simulink model "gm_minutiaeextraction_21821"  (R2018b)
settings: Solver=FixedStepDiscrete  StartTime=0.0  StopTime=10  RelTol=1e-3
undefined symbols (not defined in the file or in its folder): gray
libraries: hdlsllib x4, visionsources x1, dspmtrx3 x1
(part 7 of 7)

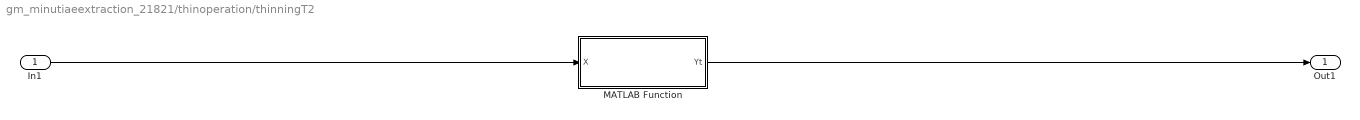
== system gm_minutiaeextraction_21821/thinoperation/thinningT2 ==
  In1 : Inport
  MATLAB Function : MATLAB Function  TreatAsAtomicUnit=on
  Out1 : Outport
  wires:
  MATLAB Function/1(Yt) -> Out1/1
  In1/1 -> MATLAB Function/1(X)

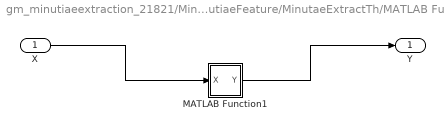
== system gm_minutiaeextraction_21821/MinutiaeFeature/MinutaeExtractTh/MATLAB Function1 ==
  X : Inport  OutDataTypeStr=boolean  PortDimensions=[128,64]  SampleTime=0.1
  MATLAB Function1 : MATLAB Function  TreatAsAtomicUnit=on
  Y : Outport
  wires:
  X/1 -> MATLAB Function1/1(X)
  MATLAB Function1/1(Y) -> Y/1

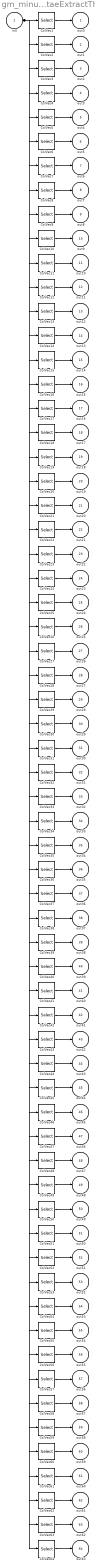
== system gm_minutiaeextraction_21821/MinutiaeFeature/MinutaeExtractTh/t ==
  in0 : Inport
  ColVec1 : Selector  NumberOfDimensions=2  IndexOptions=Select all,Index vector (dialog)  Indices=1,1  OutputSizes=1,1
  ColVec10 : Selector  NumberOfDimensions=2  IndexOptions=Select all,Index vector (dialog)  Indices=1,10  OutputSizes=1,1
  ColVec11 : Selector  NumberOfDimensions=2  IndexOptions=Select all,Index vector (dialog)  Indices=1,11  OutputSizes=1,1
  ColVec12 : Selector  NumberOfDimensions=2  IndexOptions=Select all,Index vector (dialog)  Indices=1,12  OutputSizes=1,1
  ColVec13 : Selector  NumberOfDimensions=2  IndexOptions=Select all,Index vector (dialog)  Indices=1,13  OutputSizes=1,1
  ColVec14 : Selector  NumberOfDimensions=2  IndexOptions=Select all,Index vector (dialog)  Indices=1,14  OutputSizes=1,1
  ColVec15 : Selector  NumberOfDimensions=2  IndexOptions=Select all,Index vector (dialog)  Indices=1,15  OutputSizes=1,1
  ColVec16 : Selector  NumberOfDimensions=2  IndexOptions=Select all,Index vector (dialog)  Indices=1,16  OutputSizes=1,1
  ColVec17 : Selector  NumberOfDimensions=2  IndexOptions=Select all,Index vector (dialog)  Indices=1,17  OutputSizes=1,1
  ColVec18 : Selector  NumberOfDimensions=2  IndexOptions=Select all,Index vector (dialog)  Indices=1,18  OutputSizes=1,1
  ColVec19 : Selector  NumberOfDimensions=2  IndexOptions=Select all,Index vector (dialog)  Indices=1,19  OutputSizes=1,1
  ColVec2 : Selector  NumberOfDimensions=2  IndexOptions=Select all,Index vector (dialog)  Indices=1,2  OutputSizes=1,1
  ColVec20 : Selector  NumberOfDimensions=2  IndexOptions=Select all,Index vector (dialog)  Indices=1,20  OutputSizes=1,1
  ColVec21 : Selector  NumberOfDimensions=2  IndexOptions=Select all,Index vector (dialog)  Indices=1,21  OutputSizes=1,1
  ColVec22 : Selector  NumberOfDimensions=2  IndexOptions=Select all,Index vector (dialog)  Indices=1,22  OutputSizes=1,1
  ColVec23 : Selector  NumberOfDimensions=2  IndexOptions=Select all,Index vector (dialog)  Indices=1,23  OutputSizes=1,1
  ColVec24 : Selector  NumberOfDimensions=2  IndexOptions=Select all,Index vector (dialog)  Indices=1,24  OutputSizes=1,1
  ColVec25 : Selector  NumberOfDimensions=2  IndexOptions=Select all,Index vector (dialog)  Indices=1,25  OutputSizes=1,1
  ColVec26 : Selector  NumberOfDimensions=2  IndexOptions=Select all,Index vector (dialog)  Indices=1,26  OutputSizes=1,1
  ColVec27 : Selector  NumberOfDimensions=2  IndexOptions=Select all,Index vector (dialog)  Indices=1,27  OutputSizes=1,1
  ColVec28 : Selector  NumberOfDimensions=2  IndexOptions=Select all,Index vector (dialog)  Indices=1,28  OutputSizes=1,1
  ColVec29 : Selector  NumberOfDimensions=2  IndexOptions=Select all,Index vector (dialog)  Indices=1,29  OutputSizes=1,1
  ColVec3 : Selector  NumberOfDimensions=2  IndexOptions=Select all,Index vector (dialog)  Indices=1,3  OutputSizes=1,1
  ColVec30 : Selector  NumberOfDimensions=2  IndexOptions=Select all,Index vector (dialog)  Indices=1,30  OutputSizes=1,1
  ColVec31 : Selector  NumberOfDimensions=2  IndexOptions=Select all,Index vector (dialog)  Indices=1,31  OutputSizes=1,1
  ColVec32 : Selector  NumberOfDimensions=2  IndexOptions=Select all,Index vector (dialog)  Indices=1,32  OutputSizes=1,1
  ColVec33 : Selector  NumberOfDimensions=2  IndexOptions=Select all,Index vector (dialog)  Indices=1,33  OutputSizes=1,1
  ColVec34 : Selector  NumberOfDimensions=2  IndexOptions=Select all,Index vector (dialog)  Indices=1,34  OutputSizes=1,1
  ColVec35 : Selector  NumberOfDimensions=2  IndexOptions=Select all,Index vector (dialog)  Indices=1,35  OutputSizes=1,1
  ColVec36 : Selector  NumberOfDimensions=2  IndexOptions=Select all,Index vector (dialog)  Indices=1,36  OutputSizes=1,1
  ColVec37 : Selector  NumberOfDimensions=2  IndexOptions=Select all,Index vector (dialog)  Indices=1,37  OutputSizes=1,1
  ColVec38 : Selector  NumberOfDimensions=2  IndexOptions=Select all,Index vector (dialog)  Indices=1,38  OutputSizes=1,1
  ColVec39 : Selector  NumberOfDimensions=2  IndexOptions=Select all,Index vector (dialog)  Indices=1,39  OutputSizes=1,1
  ColVec4 : Selector  NumberOfDimensions=2  IndexOptions=Select all,Index vector (dialog)  Indices=1,4  OutputSizes=1,1
  ColVec40 : Selector  NumberOfDimensions=2  IndexOptions=Select all,Index vector (dialog)  Indices=1,40  OutputSizes=1,1
  ColVec41 : Selector  NumberOfDimensions=2  IndexOptions=Select all,Index vector (dialog)  Indices=1,41  OutputSizes=1,1
  ColVec42 : Selector  NumberOfDimensions=2  IndexOptions=Select all,Index vector (dialog)  Indices=1,42  OutputSizes=1,1
  ColVec43 : Selector  NumberOfDimensions=2  IndexOptions=Select all,Index vector (dialog)  Indices=1,43  OutputSizes=1,1
  ColVec44 : Selector  NumberOfDimensions=2  IndexOptions=Select all,Index vector (dialog)  Indices=1,44  OutputSizes=1,1
  ColVec45 : Selector  NumberOfDimensions=2  IndexOptions=Select all,Index vector (dialog)  Indices=1,45  OutputSizes=1,1
  ColVec46 : Selector  NumberOfDimensions=2  IndexOptions=Select all,Index vector (dialog)  Indices=1,46  OutputSizes=1,1
  ColVec47 : Selector  NumberOfDimensions=2  IndexOptions=Select all,Index vector (dialog)  Indices=1,47  OutputSizes=1,1
  ColVec48 : Selector  NumberOfDimensions=2  IndexOptions=Select all,Index vector (dialog)  Indices=1,48  OutputSizes=1,1
  ColVec49 : Selector  NumberOfDimensions=2  IndexOptions=Select all,Index vector (dialog)  Indices=1,49  OutputSizes=1,1
  ColVec5 : Selector  NumberOfDimensions=2  IndexOptions=Select all,Index vector (dialog)  Indices=1,5  OutputSizes=1,1
  ColVec50 : Selector  NumberOfDimensions=2  IndexOptions=Select all,Index vector (dialog)  Indices=1,50  OutputSizes=1,1
  ColVec51 : Selector  NumberOfDimensions=2  IndexOptions=Select all,Index vector (dialog)  Indices=1,51  OutputSizes=1,1
  ColVec52 : Selector  NumberOfDimensions=2  IndexOptions=Select all,Index vector (dialog)  Indices=1,52  OutputSizes=1,1
  ColVec53 : Selector  NumberOfDimensions=2  IndexOptions=Select all,Index vector (dialog)  Indices=1,53  OutputSizes=1,1
  ColVec54 : Selector  NumberOfDimensions=2  IndexOptions=Select all,Index vector (dialog)  Indices=1,54  OutputSizes=1,1
  ColVec55 : Selector  NumberOfDimensions=2  IndexOptions=Select all,Index vector (dialog)  Indices=1,55  OutputSizes=1,1
  ColVec56 : Selector  NumberOfDimensions=2  IndexOptions=Select all,Index vector (dialog)  Indices=1,56  OutputSizes=1,1
  ColVec57 : Selector  NumberOfDimensions=2  IndexOptions=Select all,Index vector (dialog)  Indices=1,57  OutputSizes=1,1
  ColVec58 : Selector  NumberOfDimensions=2  IndexOptions=Select all,Index vector (dialog)  Indices=1,58  OutputSizes=1,1
  ColVec59 : Selector  NumberOfDimensions=2  IndexOptions=Select all,Index vector (dialog)  Indices=1,59  OutputSizes=1,1
  ColVec6 : Selector  NumberOfDimensions=2  IndexOptions=Select all,Index vector (dialog)  Indices=1,6  OutputSizes=1,1
  ColVec60 : Selector  NumberOfDimensions=2  IndexOptions=Select all,Index vector (dialog)  Indices=1,60  OutputSizes=1,1
  ColVec61 : Selector  NumberOfDimensions=2  IndexOptions=Select all,Index vector (dialog)  Indices=1,61  OutputSizes=1,1
  ColVec62 : Selector  NumberOfDimensions=2  IndexOptions=Select all,Index vector (dialog)  Indices=1,62  OutputSizes=1,1
  ColVec63 : Selector  NumberOfDimensions=2  IndexOptions=Select all,Index vector (dialog)  Indices=1,63  OutputSizes=1,1
  ColVec64 : Selector  NumberOfDimensions=2  IndexOptions=Select all,Index vector (dialog)  Indices=1,64  OutputSizes=1,1
  ColVec7 : Selector  NumberOfDimensions=2  IndexOptions=Select all,Index vector (dialog)  Indices=1,7  OutputSizes=1,1
  ColVec8 : Selector  NumberOfDimensions=2  IndexOptions=Select all,Index vector (dialog)  Indices=1,8  OutputSizes=1,1
  ColVec9 : Selector  NumberOfDimensions=2  IndexOptions=Select all,Index vector (dialog)  Indices=1,9  OutputSizes=1,1
  out0 : Outport
  out1 : Outport  Port=2
  out2 : Outport  Port=3
  out3 : Outport  Port=4
  out4 : Outport  Port=5
  out5 : Outport  Port=6
  out6 : Outport  Port=7
  out7 : Outport  Port=8
  out8 : Outport  Port=9
  out9 : Outport  Port=10
  out10 : Outport  Port=11
  out11 : Outport  Port=12
  out12 : Outport  Port=13
  out13 : Outport  Port=14
  out14 : Outport  Port=15
  out15 : Outport  Port=16
  out16 : Outport  Port=17
  out17 : Outport  Port=18
  out18 : Outport  Port=19
  out19 : Outport  Port=20
  out20 : Outport  Port=21
  out21 : Outport  Port=22
  out22 : Outport  Port=23
  out23 : Outport  Port=24
  out24 : Outport  Port=25
  out25 : Outport  Port=26
  out26 : Outport  Port=27
  out27 : Outport  Port=28
  out28 : Outport  Port=29
  out29 : Outport  Port=30
  out30 : Outport  Port=31
  out31 : Outport  Port=32
  out32 : Outport  Port=33
  out33 : Outport  Port=34
  out34 : Outport  Port=35
  out35 : Outport  Port=36
  out36 : Outport  Port=37
  out37 : Outport  Port=38
  out38 : Outport  Port=39
  out39 : Outport  Port=40
  out40 : Outport  Port=41
  out41 : Outport  Port=42
  out42 : Outport  Port=43
  out43 : Outport  Port=44
  out44 : Outport  Port=45
  out45 : Outport  Port=46
  out46 : Outport  Port=47
  out47 : Outport  Port=48
  out48 : Outport  Port=49
  out49 : Outport  Port=50
  out50 : Outport  Port=51
  out51 : Outport  Port=52
  out52 : Outport  Port=53
  out53 : Outport  Port=54
  out54 : Outport  Port=55
  out55 : Outport  Port=56
  out56 : Outport  Port=57
  out57 : Outport  Port=58
  out58 : Outport  Port=59
  out59 : Outport  Port=60
  out60 : Outport  Port=61
  out61 : Outport  Port=62
  out62 : Outport  Port=63
  out63 : Outport  Port=64
  wires:
  in0/1 -> ColVec1/1, ColVec2/1, ColVec3/1, ColVec4/1, ColVec5/1, ColVec6/1, ColVec7/1, ColVec8/1, ColVec9/1, ColVec10/1, ColVec11/1, ColVec12/1, ColVec13/1, ColVec14/1, ColVec15/1, ColVec16/1, ColVec17/1, ColVec18/1, ColVec19/1, ColVec20/1, ColVec21/1, ColVec22/1, ColVec23/1, ColVec24/1, ColVec25/1, ColVec26/1, ColVec27/1, ColVec28/1, ColVec29/1, ColVec30/1, ColVec31/1, ColVec32/1, ColVec33/1, ColVec34/1, ColVec35/1, ColVec36/1, ColVec37/1, ColVec38/1, ColVec39/1, ColVec40/1, ColVec41/1, ColVec42/1, ColVec43/1, ColVec44/1, ColVec45/1, ColVec46/1, ColVec47/1, ColVec48/1, ColVec49/1, ColVec50/1, ColVec51/1, ColVec52/1, ColVec53/1, ColVec54/1, ColVec55/1, ColVec56/1, ColVec57/1, ColVec58/1, ColVec59/1, ColVec60/1, ColVec61/1, ColVec62/1, ColVec63/1, ColVec64/1
  ColVec1/1 -> out0/1
  ColVec2/1 -> out1/1
  ColVec3/1 -> out2/1
  ColVec4/1 -> out3/1
  ColVec5/1 -> out4/1
  ColVec6/1 -> out5/1
  ColVec7/1 -> out6/1
  ColVec8/1 -> out7/1
  ColVec9/1 -> out8/1
  ColVec10/1 -> out9/1
  ColVec11/1 -> out10/1
  ColVec12/1 -> out11/1
  ColVec13/1 -> out12/1
  ColVec14/1 -> out13/1
  ColVec15/1 -> out14/1
  ColVec16/1 -> out15/1
  ColVec17/1 -> out16/1
  ColVec18/1 -> out17/1
  ColVec19/1 -> out18/1
  ColVec20/1 -> out19/1
  ColVec21/1 -> out20/1
  ColVec22/1 -> out21/1
  ColVec23/1 -> out22/1
  ColVec24/1 -> out23/1
  ColVec25/1 -> out24/1
  ColVec26/1 -> out25/1
  ColVec27/1 -> out26/1
  ColVec28/1 -> out27/1
  ColVec29/1 -> out28/1
  ColVec30/1 -> out29/1
  ColVec31/1 -> out30/1
  ColVec32/1 -> out31/1
  ColVec33/1 -> out32/1
  ColVec34/1 -> out33/1
  ColVec35/1 -> out34/1
  ColVec36/1 -> out35/1
  ColVec37/1 -> out36/1
  ColVec38/1 -> out37/1
  ColVec39/1 -> out38/1
  ColVec40/1 -> out39/1
  ColVec41/1 -> out40/1
  ColVec42/1 -> out41/1
  ColVec43/1 -> out42/1
  ColVec44/1 -> out43/1
  ColVec45/1 -> out44/1
  ColVec46/1 -> out45/1
  ColVec47/1 -> out46/1
  ColVec48/1 -> out47/1
  ColVec49/1 -> out48/1
  ColVec50/1 -> out49/1
  ColVec51/1 -> out50/1
  ColVec52/1 -> out51/1
  ColVec53/1 -> out52/1
  ColVec54/1 -> out53/1
  ColVec55/1 -> out54/1
  ColVec56/1 -> out55/1
  ColVec57/1 -> out56/1
  ColVec58/1 -> out57/1
  ColVec59/1 -> out58/1
  ColVec60/1 -> out59/1
  ColVec61/1 -> out60/1
  ColVec62/1 -> out61/1
  ColVec63/1 -> out62/1
  ColVec64/1 -> out63/1

== matlab function gm_minutiaeextraction_21821/MATLAB Function2 ==
  data: u input; y output
function y = fcn(u)
%#codegen
%i = rgb2gray(u);
b = u(100:227,150:213);
y = imbinarize(b);
%y = y(100:227,150:213);
%y = imbinarize(r);

== matlab function gm_minutiaeextraction_21821/thinoperation/thinningT2/MATLAB Function ==
  data: X input; Yt output
function Yt=thinningTh(X)
%img = imread ('2_4.jpg'); 
%Xr = rgb2gray(img);
%%%X = imbinarize(Xr);
%X = X(1:128,1:64);
[M,N]=size(X);
Yt = false(M,N);
Y=false(M,N,20);
Z=false(M,N,20);
Y(:,:,1)=X;
Z(:,:,1)=X;
for k=2:20
    Y(:,:,k)=Y(:,:,k-1);
    for i=2:M-1
        for j=2:N-1
            y11=Y(i-1,j-1,k);
            y12=Y(i-1,j,k);
            y13=Y(i-1,j+1,k);
            y21=Y(i,j-1,k);
            y22=Y(i,j,k);
            y23=Y(i,j+1,k);
            y31=Y(i+1,j-1,k);
            y32=Y(i+1,j,k);
            y33=Y(i+1,j+1,k);
            if y22==0
                if y11==1&&y12==1&&y13==1&&y31==0&&y32==0&&y33==0
                    Y(i,j,k)=1;
                elseif y11==1&&y13==0&&y21==1&&y23==0&&y31==1&&y33==0
                    Y(i,j,k)=1;
                elseif y11==0&&y12==0&&y13==0&&y31==1&&y32==1&&y33==1
                    Y(i,j,k)=1;
                elseif y11==0&&y13==1&&y21==0&&y23==1&&y31==0&&y33==1
                    Y(i,j,k)=1;
                elseif y12==1&&y13==1&&y21==0&&y23==1&&y32==0
                    Y(i,j,k)=1;
                elseif y11==1&&y12==1&&y21==1&&y23==0&&y32==0
                    Y(i,j,k)=1;
                elseif y12==0&&y21==1&&y23==0&&y31==1&&y21==1
                    Y(i,j,k)=1;
                elseif y12==0&&y21==0&&y23==1&&y32==1&&y33==1
                    Y(i,j,k)=1;
                    %extra
                elseif y11==0&&y12==0&&y23==1&&y31==1&&y32==1&&y33==1
                    Y(i,j,k)=1;
                end
            else
            end
        end
    end
%    Y(:,:,k)= Y(:,:,k-1);
     if Y(:,:,k)==Y(:,:,k-1)
%         break;
     end
end
Yt=Y(:,:,k);
%figure;
%imshow(Y);

== matlab function gm_minutiaeextraction_21821/MinutiaeFeature/MinutaeExtractTh/MATLAB Function1/MATLAB Function1 ==
  data: X input; Y output
function Y=minuextractT(X)
%img = imread ('101_7.tif'); 
%Xr = rgb2gray(img);
%Xt = imbinarize(img);
%X=~bwmorph(Xt,'thin',Inf);
[M,N]=size(X);
%mi(:,:)=X;
Y=false(M,N);
Y(:,:)=X;
%[M,N]=size(X);
mi=false(M,N);

for i=2:M-1
    for j=2:N-1
        % * * * y11 y12 y13
        % * @ * y21 y22 y23
        % * * * y31 y32 y33
        y11=Y(i-1,j-1);
        y12=Y(i-1,j);
        y13=Y(i-1,j+1);
        y21=Y(i,j-1);
        y22=Y(i,j);
        y23=Y(i,j+1);
        y31=Y(i+1,j-1);
        y32=Y(i+1,j);
        y33=Y(i+1,j+1);
        if y22==0
            if y11+y12+y13+y23+y33+y31+y21+y32==7
                mi(i,j)=1;
            elseif y11==0 && y12==1 && y13==0 && y21==1 && y23==1 && y31==1 && y32==0 && y33==1
                mi(i,j)=2;
            elseif y11==1 && y12==0 && y13==1 && y21==1 && y23==1 && y31==0 && y32==1 && y33==0
                mi(i,j)=2;
            elseif y11==0 && y12==1 && y13==1 && y21==1 && y23==0 && y31==0 && y32==1 && y33==1
                mi(i,j)=2;
            elseif y11==1 && y12==1 && y13==0 && y21==0 && y23==1 && y31==1 && y32==1 && y33==0
                mi(i,j)=2;
            elseif y11==1 && y12==0 && y13==1 && y21==0 && y23==0 && y31==1 && y32==1 && y33==1
                mi(i,j)=2;
            elseif y11==1 && y12==1 && y13==1 && y21==0 && y23==0 && y31==1 && y32==0 && y33==1
                mi(i,j)=2;
            elseif y11==1 && y12==0 && y13==1 && y21==0 && y23==1 && y31==1 && y32==0 && y33==1
                mi(i,j)=2;
            elseif y11==1 && y12==0 && y13==1 && y21==1 && y23==0 && y31==1 && y32==0 && y33==1
                mi(i,j)=2;
            elseif y11==0 && y12==1 && y13==0 && y21==1 && y23==1 && y31==0 && y32==1 && y33==1
                mi(i,j)=2;
            elseif y11==0 && y12==1 && y13==1 && y21==1 && y23==1 && y31==0 && y32==1 && y33==0
                mi(i,j)=2;
            elseif y11==0 && y12==1 && y13==0 && y21==1 && y23==1 && y31==1 && y32==1 && y33==0
                mi(i,j)=2;
            elseif y11==1 && y12==1 && y13==0 && y21==1 && y23==1 && y31==0 && y32==1 && y33==0
                mi(i,j)=2;
            elseif y11==1 && y12==0 && y13==1 && y21==0 && y23==0 && y31==0 && y32==1 && y33==1
                mi(i,j)=2;
            elseif y11==1 && y12==0 && y13==1 && y21==0 && y23==0 && y31==1 && y32==1 && y33==0
                mi(i,j)=2;
            elseif y11==0 && y12==1 && y13==1 && y21==0 && y23==0 && y31==1 && y32==0 && y33==1
                mi(i,j)=2;
            elseif y11==1 && y12==1 && y13==0 && y21==0 && y23==0 && y31==1 && y32==0 && y33==1
                mi(i,j)=2;
            elseif y11==1 && y12==1 && y13==0 && y21==0 && y23==1 && y31==1 && y32==0 && y33==1
                mi(i,j)=2;
            elseif y11==1 && y12==0 && y13==1 && y21==1 && y23==0 && y31==0 && y32==1 && y33==1
                mi(i,j)=2;
            elseif y11==1 && y12==0 && y13==1 && y21==0 && y23==1 && y31==1 && y32==1 && y33==0
                mi(i,j)=2;
            elseif y11==0 && y12==1 && y13==1 && y21==1 && y23==0 && y31==1 && y32==0 && y33==1
                mi(i,j)=2;
            elseif y11==1 && y12==0 && y13==1 && y21==1 && y23==0 && y31==0 && y32==0 && y33==1
                mi(i,j)=2;
            elseif y11==0 && y12==0 && y13==1 && y21==1 && y23==0 && y31==1 && y32==0 && y33==1
                mi(i,j)=2;
            elseif y11==1 && y12==0 && y13==0 && y21==0 && y23==1 && y31==1 && y32==0 && y33==1
                mi(i,j)=2;
            elseif y11==1 && y12==0 && y13==1 && y21==0 && y23==1 && y31==1 && y32==0 && y33==0
                mi(i,j)=2;
            end
        else
        end
    end
end
 Y=mi(:,:);

% %false minutiae deletion
% for M=1:300
%     for N=1:200
%         if mi(M,N)==1||mi(M,N)==2
%             d=20;
%             if M<d||M+d>300||N<d||N+d>200
%                 mi(M,N)=0;
%             else
%             end
%         else
%         end
%     end
% end
% 
% for N=1:200
%     for M=1:300
%         if mi(M,N)==1||mi(M,N)==2
%             for i=1:300
%                 for j=1:200
%                     if mi(i,j)==1||mi(i,j)==2
%                         if mi(M,N)==mi(i,j)
%                             d=10;
%                         else
%                             d=5;
%                         end
%                         a=sqrt((M-i)^2+(N-j)^2);
%                         if a<d&&a>0
%                             mi(M,N)=0;
%                             mi(i,j)=0;
%                         else
%                         end
%                     end
%                 end
%             end
%         else
%         end
%     end
% end
% figure
% hold on
% for M=1:320
%     for N=1:240
%         if mi(M,N)==1
%             a=round((M-1)/12)+1;
%             b=round((N-1)/12)+1;
%             plot(1*(N++1i*(M)),'ro','LineWidth',2)
%         elseif mi(M,N)==2
%             a=round((M-1)/12)+1;
%             b=round((N-1)/12)+1;
%             plot(1*(N++1i*(M)),'bo','LineWidth',2)
%         end
%     end
% end

%figure;imshow(img);
%figure;imshow(Xr);
%figure;imshow(Xt);
%figure;imshow(X);
%figure;imshow(Y);
